simulink model "simul_lineaire"  (R2014b)
settings: Solver=ode45  StartTime=0.0  StopTime=10.0  RelTol=1e-3
values from neighbouring files (symbols this model uses):
  A = sym('A', [13 13])    [equation_etat_courants.m]
  B = sym('B', [13 3])    [equation_etat_courants.m]
  C = sym('B', [7 13])    [equation_etat_courants.m]
  D = zeros(7, 3)    [equation_etat_courants.m]
  U = [Va Vb Vc]    [equation_etat_courants.m]
libraries: simulink x1
settings Model: Creator=Eric  LastModifiedBy=Eric
settings OptimizationCC: UseDivisionForNetSlopeComputation=off  SimCompilerOptimization=off
settings DebuggingCC: FrameProcessingCompatibilityMsg=error  AllowSymbolicDim=off
settings RTWCC: RTWCompilerOptimization=off
settings ConfigComp: CovMetricSettings=dw  CovHtmlReporting=on  CovSaveCumulativeToWorkspaceVar=on  CovSaveSingleToWorkspaceVar=on  CovModelRefEnable=Off  CovExternalEMLEnable=off  CovSFcnEnable=off

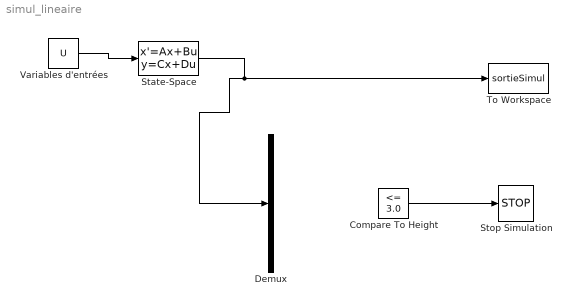
== system simul_lineaire ==
  Compare To Height : simulink/Logic and Bit Operations/Compare To Constant  relop=<=  const=3.0  OutDataTypeStr=boolean
  Demux : Demux  Outputs=7
  State-Space : StateSpace  A=A  B=B  C=C  D=D  X0=0
  Stop Simulation : Stop
  To Workspace : ToWorkspace  VariableName=sortieSimul  SaveFormat=Timeseries  SampleTime=-1
  Variables d'entrées : Constant  Value=U
  wires:
  State-Space/1 -> To Workspace/1, Demux/1
  Variables d'entrées/1 -> State-Space/1
  Compare To Height/1 -> Stop Simulation/1
